simulink model "PWPF_model"  (R2016b)
settings: Solver=VariableStepAuto  StartTime=0.0  StopTime=100  RelTol=1e-3
settings Model: Creator=Reza  LastModifiedBy=Reza

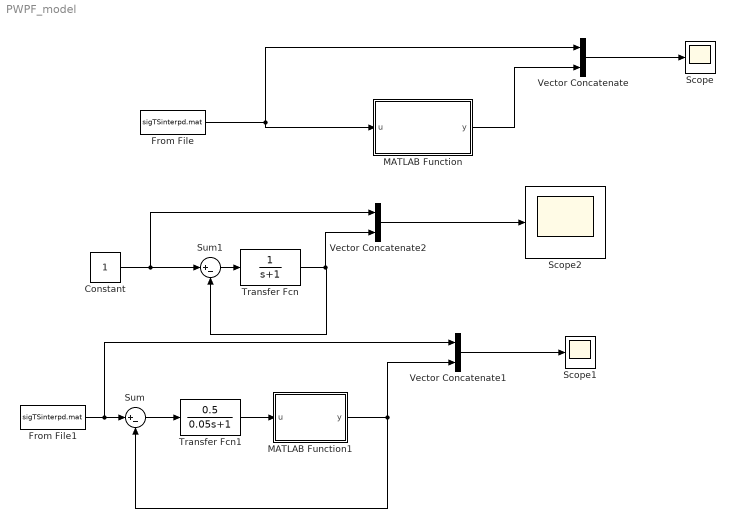
== system PWPF_model ==
  Constant : Constant
  From File : FromFile  FileName=sigTSinterpd.mat  SampleTime=0
  From File1 : FromFile  FileName=sigTSinterpd.mat  SampleTime=0
  MATLAB Function : MATLAB Function  TreatAsAtomicUnit=on
  MATLAB Function1 : MATLAB Function  TreatAsAtomicUnit=on
  Scope : Scope
  Scope1 : Scope
  Scope2 : Scope
  Sum : Sum  Inputs=|+-
  Sum1 : Sum  Inputs=|+-
  Transfer Fcn : TransferFcn  Denominator=[1 1]
  Transfer Fcn1 : TransferFcn  Numerator=[0.5]  Denominator=[0.05 1]
  Vector Concatenate : Concatenate
  Vector Concatenate1 : Concatenate
  Vector Concatenate2 : Concatenate
  wires:
  MATLAB Function/1(y) -> Vector Concatenate/2
  From File/1 -> Vector Concatenate/1, MATLAB Function/1(u)
  Vector Concatenate/1 -> Scope/1
  From File1/1 -> Sum/1, Vector Concatenate1/1
  Vector Concatenate1/1 -> Scope1/1
  Transfer Fcn1/1 -> MATLAB Function1/1(u)
  MATLAB Function1/1(y) -> Sum/2, Vector Concatenate1/2
  Sum/1 -> Transfer Fcn1/1
  Constant/1 -> Vector Concatenate2/1, Sum1/1
  Transfer Fcn/1 -> Sum1/2, Vector Concatenate2/2
  Vector Concatenate2/1 -> Scope2/1
  Sum1/1 -> Transfer Fcn/1

== matlab function PWPF_model/MATLAB Function1 ==
  data: u input; y output
function y = fcn(u)
persistent us
Uout = 0.0625;
Uon = Uout*0.4;
Uoff = Uon*0.5;

if isempty(us) 
    us = u;
end

if( abs(u) < Uoff )
    us = 0;
end

if( abs(u) > Uon )
    if(u > Uon)
        us = Uout;
    else
        us = -Uout;
    end
end

y = us;

== matlab function PWPF_model/MATLAB Function ==
  data: u input; y output
function y = fcn(u)
persistent us
lt = 0.01;
ht = 0.04;
Uout = 0.0625;

if isempty(us) 
    us = u;
end

if( abs(u) < lt )
    us = 0;
end

if( abs(u) > ht )
    if(u > ht)
        us = Uout;
    else
        us = -Uout;
    end
end

y = us;
